simulink model "ANCbyRecursive"  (R2024a)
settings: Solver=VariableStepAuto  StartTime=0.0  StopTime=inf  RelTol=1e-3
settings Model: Creator=chenxinzhang  LastModifiedBy=chenxinzhang

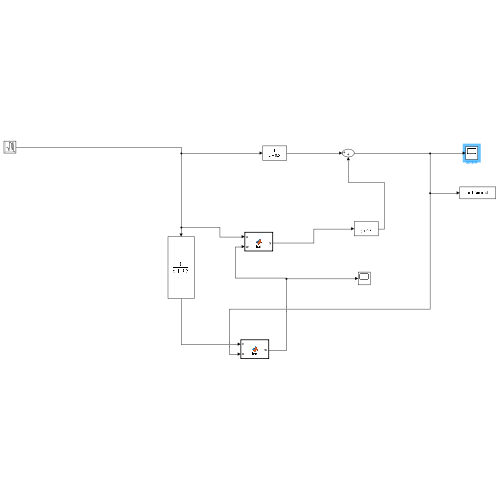
[thumbnail: Simulink's stored preview of the top-level diagram]
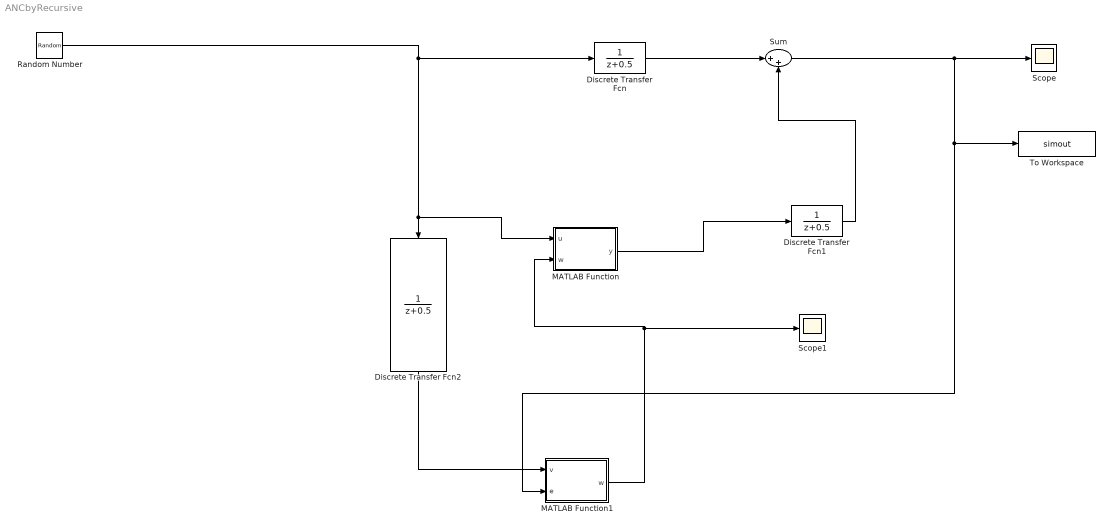
== system ANCbyRecursive ==
  Discrete Transfer Fcn : DiscreteTransferFcn  Numerator=[0 1]
  Discrete Transfer Fcn1 : DiscreteTransferFcn  Numerator=[0 1]
  Discrete Transfer Fcn2 : DiscreteTransferFcn  Numerator=[0 1]
  MATLAB Function : MATLAB Function  TreatAsAtomicUnit=on
  MATLAB Function1 : MATLAB Function  TreatAsAtomicUnit=on
  Random Number : RandomNumber  SampleTime=0.1
  Scope : Scope
  Scope1 : Scope
  Sum : Sum  Inputs=|++
  To Workspace : ToWorkspace  VariableName=simout  SaveFormat=Timeseries  SampleTime=-1
  wires:
  Discrete Transfer Fcn/1 -> Sum/1
  Discrete Transfer Fcn2/1 -> MATLAB Function1/1(v)
  Sum/1 -> To Workspace/1, MATLAB Function1/2(e), Scope/1
  MATLAB Function1/1(w) -> Scope1/1, MATLAB Function/2(w)
  MATLAB Function/1(y) -> Discrete Transfer Fcn1/1
  Discrete Transfer Fcn1/1 -> Sum/2
  Random Number/1 -> Discrete Transfer Fcn2/1, MATLAB Function/1(u), Discrete Transfer Fcn/1

== matlab function ANCbyRecursive/MATLAB Function ==
  data: u input; y output; w input
function y = fcn(u, w)
%#codegen
persistent xbuf

if isempty(xbuf)
    xbuf = zeros(1,8);
end

xbuf(2:8) = xbuf(1:7);
xbuf(1) = u;

y = w * xbuf.';

if ~isfinite(y)
    y = 0;
elseif y > 1e3
    y = 1e3;
elseif y < -1e3
    y = -1e3;
end

== matlab function ANCbyRecursive/MATLAB Function1 ==
  data: v input; w output; e input
function w = fcn(v, e)
%#codegen
persistent wbuf vbuf P
N = 8;
delta = 100;

if isempty(wbuf)
    wbuf = zeros(N,1);
end

if isempty(vbuf)
    vbuf = zeros(N,1);
end

if isempty(P)
    P = delta * eye(N);
end

vbuf(2:N) = vbuf(1:N-1);
vbuf(1) = v;

den = 0.0037+ vbuf' * P * vbuf;
K = (P * vbuf) / den;

eps = -e - vbuf' * wbuf;

wbuf = wbuf + K * eps;

P = (eye(N) - K * vbuf') * P;

for i = 1:N
    if ~isfinite(wbuf(i))
        wbuf(i) = 0;
    end
end

w = wbuf.';
